simulink model "test_speed_ctr"  (R2023a)
settings: Solver=VariableStepAuto  StartTime=0.0  StopTime=10.0  RelTol=1e-3
undefined symbols (not defined in the file): Drive
libraries: robotlib x6, simulink x2
settings Model: Creator=gptp  LastModifiedBy=gptp

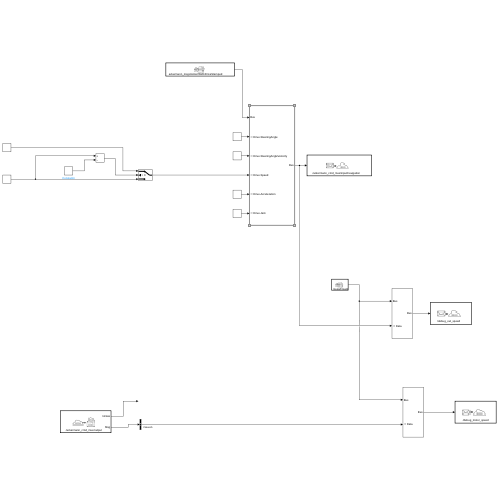
[thumbnail: Simulink's stored preview of the top-level diagram]
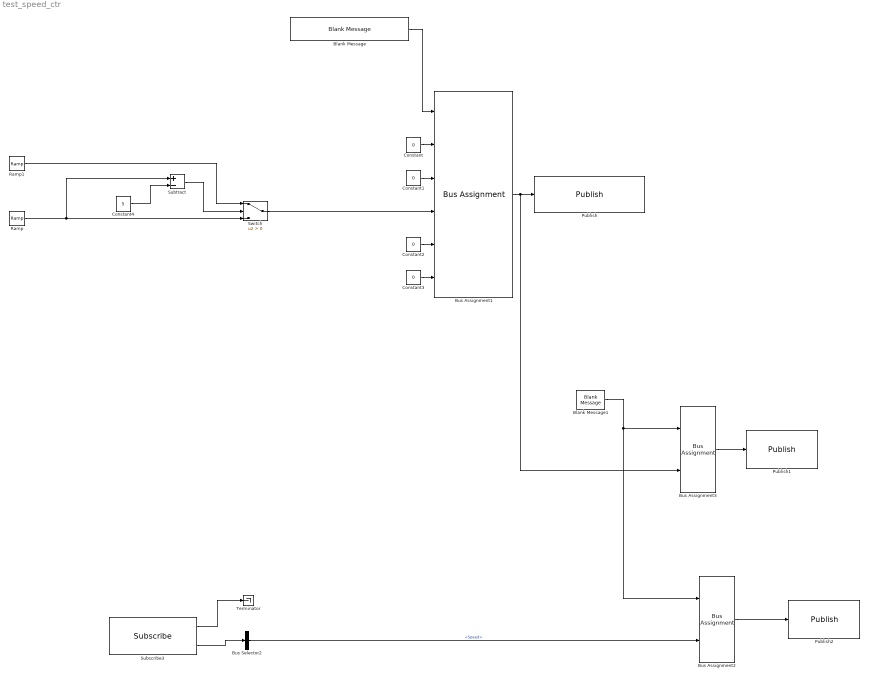
== system test_speed_ctr ==
  Blank Message : robotlib/Blank Message  messageClass=Message  entityType=ackermann_msgs/AckermannDriveStamped  messageType=ackermann_msgs/AckermannDriveStamped  SampleTime=inf  legacyBusStruct=off
  Blank Message1 : robotlib/Blank Message  messageClass=Message  entityType=std_msgs/Float32  messageType=std_msgs/Float32  SampleTime=inf  legacyBusStruct=off
  Bus Assignment1 : BusAssignment  AssignedSignals=Drive.SteeringAngle,Drive.SteeringAngleVelocity,Drive.Speed,Drive.Acceleration,Drive.Jerk
  Bus Assignment2 : BusAssignment  AssignedSignals=Data
  Bus Assignment3 : BusAssignment  AssignedSignals=Data
  Bus Selector2 : BusSelector  OutputSignals=Drive.Speed
  Constant{,1..3} (4 alike) : Constant  Value=0  OutDataTypeStr=single
  Constant4 : Constant  Value=5
  Publish : robotlib/Publish  topicSource=Specify your own  topic=/ackermann_cmd_mux/input/navigation  messageType=ackermann_msgs/AckermannDriveStamped  legacyBusStruct=off  messageQueueLength=1
  Publish1 : robotlib/Publish  topicSource=Specify your own  topic=/debug_out_speed  messageType=std_msgs/Float32  legacyBusStruct=off  messageQueueLength=1
  Publish2 : robotlib/Publish  topicSource=Specify your own  topic=/debug_motor_speed  messageType=std_msgs/Float32  legacyBusStruct=off  messageQueueLength=1
  Ramp : simulink/Sources/Ramp  slope=1  start=0  InitialOutput=0
  Ramp1 : simulink/Sources/Ramp  slope=-1  start=0  InitialOutput=10
  Subscribe3 : robotlib/Subscribe  topicSource=Specify your own  topic=/ackermann_cmd_mux/output  messageType=ackermann_msgs/AckermannDriveStamped  SampleTime=-1  legacyBusStruct=off  messageQueueLength=10
  Subtract : Sum  Inputs=+-
  Switch : Switch  Criteria=u2 > Threshold  SaturateOnIntegerOverflow=off  InputSameDT=off
  Terminator : Terminator
  wires:
  Subscribe3/2 -> Bus Selector2/1
  Bus Selector2/1 -> Bus Assignment2/2  "<Speed>"
  Subscribe3/1 -> Terminator/1
  Bus Assignment2/1 -> Publish2/1
  Blank Message1/1 -> Bus Assignment3/1, Bus Assignment2/1
  Bus Assignment1/1 -> Bus Assignment3/2, Publish/1
  Constant2/1 -> Bus Assignment1/5
  Blank Message/1 -> Bus Assignment1/1
  Constant/1 -> Bus Assignment1/2
  Constant3/1 -> Bus Assignment1/6
  Constant1/1 -> Bus Assignment1/3
  Bus Assignment3/1 -> Publish1/1
  Ramp/1 -> Subtract/1, Switch/3
  Constant4/1 -> Subtract/2
  Subtract/1 -> Switch/2
  Switch/1 -> Bus Assignment1/4
  Ramp1/1 -> Switch/1
